simulink model "testTriggerToPulse"  (R2014a)
settings: Solver=FixedStepDiscrete  StartTime=0.0  StopTime=Inf  FixedStep=0.001  RelTol=1e-3
libraries: dspswit3 x2, libTrigger x2, dspmathops x1, simulink x1
settings Model: BufferReuse=off  Creator=Dan  LastModifiedBy=djoshea
settings SolverCC: EnableConcurrentExecution=on
settings OptimizationCC: BlockReduction=off  OptimizeBlockIOStorage=off  BufferReuse=off  GlobalBufferReuse=off  ExpressionFolding=off  LocalBlockOutputs=off
settings HardwareCC: ProdIntDivRoundTo=Zero  ProdEndianess=LittleEndian  ProdHWDeviceType=Generic->32-bit x86 compatible
settings RTWCC: SystemTargetFile=slrt.tlc  TemplateMakefile=slrt_default_tmf  Description=Simulink Real-Time  ProcessScript=slrt_make_rtw_hook  RTWCompilerOptimization=On
settings TargetCC: CodeReplacementLibrary=XPC_BLAS  ParMdlRefBuildCompliant=on  ConcurrentExecutionCompliant=on  MatFileLogging=on  EnableShiftOperators=on  MATLABClassNameForMDSCustomization=xpcAperiodicCustomization

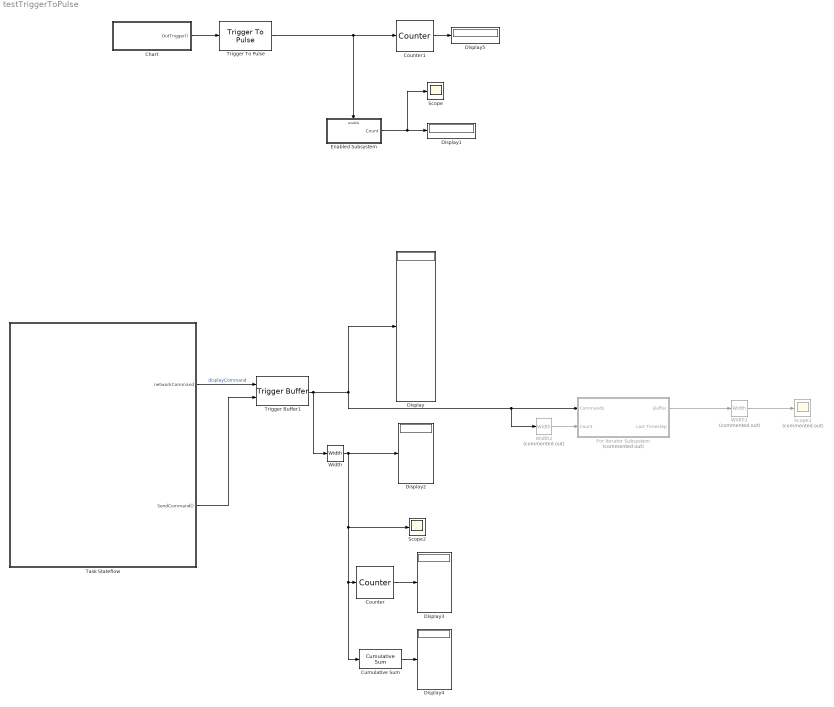
== system testTriggerToPulse ==
  Chart : Stateflow chart  TreatAsAtomicUnit=on
  Counter : dspswit3/Counter  Direction=Up  CountEvent=Non-zero sample  CounterSize=32 bits  MaxCount=255  InitialCount=0  Output=Count  HitValue=32  ResetInput=off  SamplesPerFrame=1  Ts=1  CntDtype=uint32  HitDtype=Logical
  Counter1 : dspswit3/Counter  Direction=Up  CountEvent=Non-zero sample  CounterSize=32 bits  MaxCount=255  InitialCount=0  Output=Count  HitValue=32  ResetInput=off  SamplesPerFrame=1  Ts=1  CntDtype=uint32  HitDtype=Logical
  Cumulative Sum : dspmathops/Cumulative Sum  dim=Channels (running sum)  InputProcessing=Columns as channels (frame based)  reset_popup=None  outputDataTypeStr=Inherit: Same as accumulator  outputLastDataTypeStr=Inherit: Same as accumulator  outputMin=[]  outputMax=[]  roundingMode=Floor  overflowMode=off
  Display{,1..5} (6 alike) : Display
  Enabled Subsystem : Subsystem  TreatAsAtomicUnit=on
  For Iterator Subsystem : Subsystem  Commented=on  TreatAsAtomicUnit=on
  Scope : Scope
  Scope1 : Scope  Commented=on
      settings: TimeRange=10000
  Scope2 : Scope
      settings: TimeRange=10000  SaveName=ScopeData2
  Task Stateflow : Stateflow chart  TreatAsAtomicUnit=on
  Trigger Buffer1 : libTrigger/Trigger Buffer  bufferSize=100
  Trigger To Pulse : libTrigger/Trigger To Pulse
  Width : Width  DataType=uint32
  Width1 : Width  Commented=on  DataType=uint32
  Width2 : Width  Commented=on  DataType=uint32
  wires:
  Enabled Subsystem/1(Count) -> Scope/1, Display1/1
  Trigger To Pulse/1 -> Counter1/1, Enabled Subsystem/Enable
  Chart/1(OutTrigger()) -> Trigger To Pulse/1
  Task Stateflow/1(networkCommand) -> Trigger Buffer1/1  "displayCommand"
  Task Stateflow/2(SendCommand()) -> Trigger Buffer1/2
  Trigger Buffer1/1 -> Width/1, Width2/1, For Iterator Subsystem/1(Commands), Display/1
  Width/1 -> Display2/1, Scope2/1, Cumulative Sum/1, Counter/1
  Counter/1 -> Display3/1
  Cumulative Sum/1 -> Display4/1
  Counter1/1 -> Display5/1
  For Iterator Subsystem/1(Buffer) -> Width1/1
  Width1/1 -> Scope1/1
  Width2/1 -> For Iterator Subsystem/2(Count)

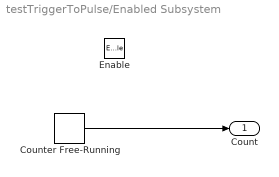
== system testTriggerToPulse/Enabled Subsystem ==
  Enable : EnablePort
  Counter Free-Running : simulink/Sources/Counter Free-Running  NumBits=16  tsamp=-1
  Count : Outport
  wires:
  Counter Free-Running/1 -> Count/1

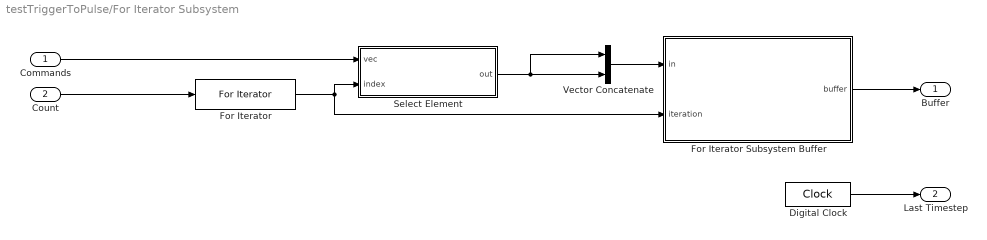
== system testTriggerToPulse/For Iterator Subsystem ==
  Commands : Inport
  Count : Inport  Port=2
  Digital Clock : DigitalClock
  For Iterator : ForIterator  ResetStates=reset  IterationSource=external
  For Iterator Subsystem Buffer : MATLAB Function  TreatAsAtomicUnit=on  mask(For Iterator Subsystem Buffer){bufferSize=100}
      mask prompts: bufferSize "Maximum Iterations"
      mask help: This block concatenates the vector inputs it receives during each iteration of a For Iterator Subsystem.
  Select Element : MATLAB Function  TreatAsAtomicUnit=on
  Vector Concatenate : Concatenate
  Buffer : Outport
      settings: VarSizeSig=Yes
  Last Timestep : Outport  Port=2
      settings: VarSizeSig=Yes
  wires:
  For Iterator Subsystem Buffer/1(buffer) -> Buffer/1
  Commands/1 -> Select Element/1(vec)
  Vector Concatenate/1 -> For Iterator Subsystem Buffer/1(in)
  Select Element/1(out) -> Vector Concatenate/2, Vector Concatenate/1
  Count/1 -> For Iterator/1
  For Iterator/1 -> Select Element/2(index), For Iterator Subsystem Buffer/2(iteration)
  Digital Clock/1 -> Last Timestep/1

== stateflow chart testTriggerToPulse/Task Stateflow ==
  state TaskControl [parallel]
    settings: executionOrder=1
    state Wait
    state Sending4_2
      en:
      networkCommand = 2;
      send(SendCommand);
    state Sending0
      en:
      networkCommand = 5;
      send(SendCommand);
      networkCommand = 6;
      send(SendCommand);
    state Sending4
      en:
      networkCommand = 1;
      send(SendCommand);
    state Sending1
      en:
      networkCommand = 1;
      send(SendCommand);
      networkCommand = 2;
      send(SendCommand);
      networkCommand = 3;
      send(SendCommand);
    state Sending2
      en:
      networkCommand = 1;
      send(SendCommand);
      networkCommand = 2;
      send(SendCommand);
      networkCommand = 3;
      send(SendCommand);
      networkCommand = 1;
      send(SendCommand);
      networkCommand = 2;
      send(SendCommand);
      networkCommand = 3;
      send(SendCommand);
      networkCommand = 1;
      send(SendCommand);
      networkCommand = 2;
      send(SendCommand);
      networkCommand = 3;
      send(SendCommand);
    (default) -> Wait
    Sending4_2 -> Sending0 : after(1000, tick)
    Wait -> Sending0 : after(1000, tick)
    Sending4 -> Sending4_2 : after(1000, tick)
    Sending2 -> Sending4 : after(1000, tick)
    Sending0 -> Sending1 : after(1000, tick)
    Sending1 -> Sending2 : after(1000, tick)
  data: networkCommand output uint16 size=1
  events: SendCommand output FUNCTION_CALL_EVENT

== matlab function testTriggerToPulse/For Iterator Subsystem/Select Element ==
  data: out output size=1; vec input; index input size=1
function out = selectElement(vec, index)
%#codegen

if index >= 1 && index <= numel(vec)
    out = vec(index);
else
    out = zeros(1, 1, 'like', vec);
end


end

== stateflow chart testTriggerToPulse/Chart ==
  state Send
    en:
    send(OutTrigger);
  state Wait
  Send -> Wait
  Wait -> Send : after(1000, tick)
  (default) -> Wait
  events: OutTrigger output FUNCTION_CALL_EVENT

== matlab function testTriggerToPulse/For Iterator Subsystem/For Iterator Subsystem Buffer ==
  data: buffer output size=bufferSize; in input; iteration input; bufferSize parameter uint32 size=1
function buffer = appendToBuffer(in, iteration, bufferSize)
%#codegen

% generated by BusSerialize.generateCoderVarsizeStatementsForBus('TestForBus', 'pBus');
coder.varsize('pBuffer', bufferSize, true);

persistent pBuffer;
if isempty(pBuffer) || uint32(iteration) == uint32(1)
    pBuffer = in(:);
elseif numel(pBuffer) + numel(in) < bufferSize
    pBuffer = [pBuffer; in(:)];
end

buffer = pBuffer;

end
